simulink model "topfft"  (Simulink 7.6)
settings: Solver=FixedStepDiscrete  StartTime=0.0  StopTime=800  RelTol=1e-3
InitFcn:
  | %% DSPBuilder Start
  | alt_dspbuilder_update_model(bdroot)
  | %% DSPBuilder End
undefined symbols (not defined in the file): DSPBuilder_topfft_import, fft_stream
libraries: allblocks_alteradspbuilder2 x18, dspsrcs4 x4, simulink x3, megacorefunctions_alteradspbuilder2 x1
settings Model: Creator=lkong  LastModifiedBy=akarapet
settings OptimizationCC: InlineInvariantSignals=on  InitFltsAndDblsToZero=on
settings DebuggingCC: SaveWithParameterizedLinksMsg=none  SignalResolutionControl=TryResolveAllWithWarning  SolverPrmCheckMsg=none  MultiTaskDSMMsg=warning  MultiTaskCondExecSysMsg=none  StrictBusMsg=Warning
settings HardwareCC: TargetUnknown=on
settings RTWCC: IncludeERTFirstTime=on
settings GRTTargetCC: TargetFcnLib=ansi_tfl_tmw.mat

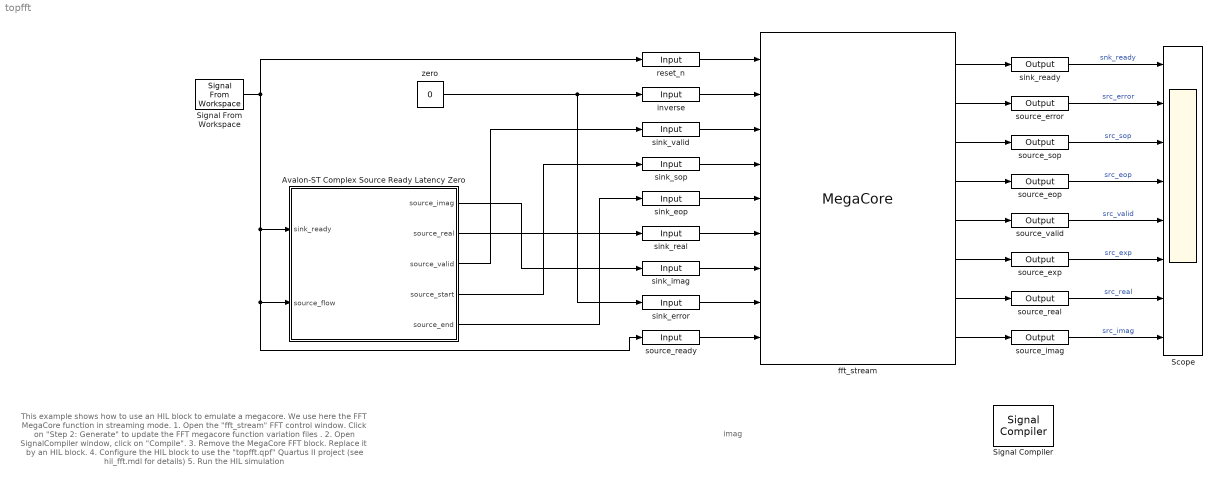
== system topfft ==
  note: imag
  note: This example shows how to use an HIL block to emulate a megacore.
      | We use here the FFT MegaCore function in streaming mode.
      | 1. Open the "fft_stream" FFT control window. Click on "Step 2: Generate" to update the FFT megacore function variation files .
      | 2. Open SignalCompiler window, click on "Compile".
      | 3. Remove the MegaCore FFT block. Replace it by an HIL block.
      | 4. Configure the HIL block to use the "topfft.qpf" Quartus II project (see hil_fft.mdl for details)
      | 5. Run the HIL simulation
  Avalon-ST Complex Source Ready Latency Zero : Subsystem  mask{datastring=[1:32], sopstring=[1 zeros(1,63)], eopstring=[zeros(1,63) 1], finaloption=Cyclic Repetition}
      mask prompts: datastring "Complex Data"; sopstring "Start of Packet"; eopstring "End of Packet"; finaloption "Form output after final data by"
      mask StyleString: edit,edit,edit,popup(Cyclic Repetition)
      mask Display:
      | port_label('input',1,'sink_ready');
      | port_label('input',2,'source_flow');
      | 
      | port_label('output',1,'source_imag');
      | port_label('output',2,'source_real');
      | port_label('output',3,'source_valid');
      | port_label('output',4,'source_start');
      | port_label('output',5,'source_end');
      | 
      | disp(&1);
  Scope : Scope  NumInputPorts=8
      settings: TimeRange=800  YMin=0~0~-1~-4~-20~-10~0~0  YMax=1~1~1~0~30~70~1~1
  Signal Compiler : allblocks_alteradspbuilder2/Signal Compiler  DeviceFamily=Cyclone III  DeviceName=EP3C120F780C7  EnableSignalTap=off  SignalTapDepth=128  UseBoardBlock=off  StpUseDefaultClock=on  StpClock=Clock  ExportDir=/data/akarapet/qshell_linux64_test/p4/dsp_builder/dsp_builder2/Documentation/DesignExamples/Tutorials/HIL/FFT
  Signal From Workspace : dspsrcs4/Signal From Workspace  SystemSampleTime=-1  X=[0 1]  Ts=1  nsamps=1  OutputAfterFinalValue=Holding final value  ignoreOrWarnInputAndFrameLengths=off
  fft_stream : megacorefunctions_alteradspbuilder2/MegaCore  entityName=fft_stream_import  inNames=reset_n inverse sink_valid sink_sop sink_eop sink_real sink_imag sink_error source_ready  inBwls="1   1   1   1   1  16  16   2   1"  inBwrs="0  0  0  0  0  0  0  0  0"  inTypes=b b b b b s s s b  inDelayed="0  1  1  1  1  1  1  1  1"  outNames=sink_ready source_error source_sop source_eop source_valid source_exp source_real source_imag  outBwls="1   2   1   1   1   6  16  16"  outBwrs="0  0  0  0  0  0  0  0"  outTypes=b s b b b s s s  xmlmapfile=/data/akarapet/qshell_linux64_test/acds/quartus/dsp_builder/lib/SimgenCMap.xml  is_megacore=on  use_dynamic_feedthrough_data=on  use_alphabetical_port_ordering=off  vofile=DSPBuilder_topfft_import/fft_stream.vo  n_input_port=9  n_output_port=8  core_dir=/data/akarapet/qshell_linux64_test/acds/ip/altera/fft/lib/ip_toolbench  core_name=fft  clockname=clk  flow_dir=/data/akarapet/qshell_linux64_test/acds/ip/altera/fft/lib/../../common/ip_toolbench/v1.3.0/bin  NewVariation=off  VhdlVariationDate=19-Jun-2013 09:53:44  VhdlVariationName=/data/akarapet/qshell_linux64_test/p4/dsp_builder/dsp_builder2/Documentation/DesignExamples/Tutorials/HIL/FFT/DSPBuilder_topfft_import/fft_stream.vhd  use_systemC_model=off  wizard=fft  inptype=bbbbbsssb  outptype=bsbbbsss  allowFloatingPointOverride=off
  inverse : allblocks_alteradspbuilder2/Input  iofile=/data/akarapet/qshell_linux64_test/p4/dsp_builder/dsp_builder2/Documentation/DesignExamples/Tutorials/HIL/FFT/tb_topfft/topfft_inverse.salt  BusType=Single Bit  bwl=1  bwr=0  SpecifyClock=off  PORTTYPE=Input  externalType=Inferred  allowFloatingPointOverride=on  logOutputs=off
  reset_n : allblocks_alteradspbuilder2/Input  iofile=/data/akarapet/qshell_linux64_test/p4/dsp_builder/dsp_builder2/Documentation/DesignExamples/Tutorials/HIL/FFT/tb_topfft/topfft_reset%5Fn.salt  BusType=Single Bit  bwl=1  bwr=0  SpecifyClock=off  PORTTYPE=Input  externalType=Inferred  allowFloatingPointOverride=on  logOutputs=off
  sink_eop : allblocks_alteradspbuilder2/Input  iofile=/data/akarapet/qshell_linux64_test/p4/dsp_builder/dsp_builder2/Documentation/DesignExamples/Tutorials/HIL/FFT/tb_topfft/topfft_sink%5Feop.salt  BusType=Single Bit  bwl=1  bwr=0  SpecifyClock=off  PORTTYPE=Input  externalType=Inferred  allowFloatingPointOverride=on  logOutputs=off
  sink_error : allblocks_alteradspbuilder2/Input  iofile=/data/akarapet/qshell_linux64_test/p4/dsp_builder/dsp_builder2/Documentation/DesignExamples/Tutorials/HIL/FFT/tb_topfft/topfft_sink%5Ferror.salt  BusType=Signed Integer  bwl=2  bwr=0  SpecifyClock=off  PORTTYPE=Input  externalType=Inferred  allowFloatingPointOverride=on  logOutputs=off
  sink_imag : allblocks_alteradspbuilder2/Input  iofile=/data/akarapet/qshell_linux64_test/p4/dsp_builder/dsp_builder2/Documentation/DesignExamples/Tutorials/HIL/FFT/tb_topfft/topfft_sink%5Fimag.salt  BusType=Signed Integer  bwl=16  bwr=0  SpecifyClock=off  PORTTYPE=Input  externalType=Inferred  allowFloatingPointOverride=on  logOutputs=off
  sink_ready : allblocks_alteradspbuilder2/Output  iofile=/data/akarapet/qshell_linux64_test/p4/dsp_builder/dsp_builder2/Documentation/DesignExamples/Tutorials/HIL/FFT/tb_topfft/topfft_sink%5Fready.capture  BusType=Single Bit  bwl=1  bwr=0  externalType=Inferred  PORTTYPE=Output  allowFloatingPointOverride=on  logOutputs=off
  sink_real : allblocks_alteradspbuilder2/Input  iofile=/data/akarapet/qshell_linux64_test/p4/dsp_builder/dsp_builder2/Documentation/DesignExamples/Tutorials/HIL/FFT/tb_topfft/topfft_sink%5Freal.salt  BusType=Signed Integer  bwl=16  bwr=0  SpecifyClock=off  PORTTYPE=Input  externalType=Inferred  allowFloatingPointOverride=on  logOutputs=off
  sink_sop : allblocks_alteradspbuilder2/Input  iofile=/data/akarapet/qshell_linux64_test/p4/dsp_builder/dsp_builder2/Documentation/DesignExamples/Tutorials/HIL/FFT/tb_topfft/topfft_sink%5Fsop.salt  BusType=Single Bit  bwl=1  bwr=0  SpecifyClock=off  PORTTYPE=Input  externalType=Inferred  allowFloatingPointOverride=on  logOutputs=off
  sink_valid : allblocks_alteradspbuilder2/Input  iofile=/data/akarapet/qshell_linux64_test/p4/dsp_builder/dsp_builder2/Documentation/DesignExamples/Tutorials/HIL/FFT/tb_topfft/topfft_sink%5Fvalid.salt  BusType=Single Bit  bwl=1  bwr=0  SpecifyClock=off  PORTTYPE=Input  externalType=Inferred  allowFloatingPointOverride=on  logOutputs=off
  source_eop : allblocks_alteradspbuilder2/Output  iofile=/data/akarapet/qshell_linux64_test/p4/dsp_builder/dsp_builder2/Documentation/DesignExamples/Tutorials/HIL/FFT/tb_topfft/topfft_source%5Feop.capture  BusType=Single Bit  bwl=1  bwr=0  externalType=Inferred  PORTTYPE=Output  allowFloatingPointOverride=on  logOutputs=off
  source_error : allblocks_alteradspbuilder2/Output  iofile=/data/akarapet/qshell_linux64_test/p4/dsp_builder/dsp_builder2/Documentation/DesignExamples/Tutorials/HIL/FFT/tb_topfft/topfft_source%5Ferror.capture  BusType=Signed Integer  bwl=2  bwr=0  externalType=Inferred  PORTTYPE=Output  allowFloatingPointOverride=on  logOutputs=off
  source_exp : allblocks_alteradspbuilder2/Output  iofile=/data/akarapet/qshell_linux64_test/p4/dsp_builder/dsp_builder2/Documentation/DesignExamples/Tutorials/HIL/FFT/tb_topfft/topfft_source%5Fexp.capture  BusType=Signed Integer  bwl=6  bwr=0  externalType=Inferred  PORTTYPE=Output  allowFloatingPointOverride=on  logOutputs=off
  source_imag : allblocks_alteradspbuilder2/Output  iofile=/data/akarapet/qshell_linux64_test/p4/dsp_builder/dsp_builder2/Documentation/DesignExamples/Tutorials/HIL/FFT/tb_topfft/topfft_source%5Fimag.capture  BusType=Signed Integer  bwl=16  bwr=0  externalType=Inferred  PORTTYPE=Output  allowFloatingPointOverride=on  logOutputs=off
  source_ready : allblocks_alteradspbuilder2/Input  iofile=/data/akarapet/qshell_linux64_test/p4/dsp_builder/dsp_builder2/Documentation/DesignExamples/Tutorials/HIL/FFT/tb_topfft/topfft_source%5Fready.salt  BusType=Single Bit  bwl=1  bwr=0  SpecifyClock=off  PORTTYPE=Input  externalType=Inferred  allowFloatingPointOverride=on  logOutputs=off
  source_real : allblocks_alteradspbuilder2/Output  iofile=/data/akarapet/qshell_linux64_test/p4/dsp_builder/dsp_builder2/Documentation/DesignExamples/Tutorials/HIL/FFT/tb_topfft/topfft_source%5Freal.capture  BusType=Signed Integer  bwl=16  bwr=0  externalType=Inferred  PORTTYPE=Output  allowFloatingPointOverride=on  logOutputs=off
  source_sop : allblocks_alteradspbuilder2/Output  iofile=/data/akarapet/qshell_linux64_test/p4/dsp_builder/dsp_builder2/Documentation/DesignExamples/Tutorials/HIL/FFT/tb_topfft/topfft_source%5Fsop.capture  BusType=Single Bit  bwl=1  bwr=0  externalType=Inferred  PORTTYPE=Output  allowFloatingPointOverride=on  logOutputs=off
  source_valid : allblocks_alteradspbuilder2/Output  iofile=/data/akarapet/qshell_linux64_test/p4/dsp_builder/dsp_builder2/Documentation/DesignExamples/Tutorials/HIL/FFT/tb_topfft/topfft_source%5Fvalid.capture  BusType=Single Bit  bwl=1  bwr=0  externalType=Inferred  PORTTYPE=Output  allowFloatingPointOverride=on  logOutputs=off
  zero : Constant  Value=0
  wires:
  zero/1 -> sink_error/1, inverse/1
  sink_imag/1 -> fft_stream/7
  sink_real/1 -> fft_stream/6
  inverse/1 -> fft_stream/2
  sink_sop/1 -> fft_stream/4
  fft_stream/4 -> source_eop/1
  fft_stream/2 -> source_error/1
  fft_stream/6 -> source_exp/1
  fft_stream/8 -> source_imag/1
  source_eop/1 -> Scope/4  "src_eop"
  source_error/1 -> Scope/2  "src_error"
  source_exp/1 -> Scope/6  "src_exp"
  source_imag/1 -> Scope/8  "src_imag"
  source_real/1 -> Scope/7  "src_real"
  source_sop/1 -> Scope/3  "src_sop"
  source_valid/1 -> Scope/5  "src_valid"
  sink_valid/1 -> fft_stream/3
  fft_stream/3 -> source_sop/1
  fft_stream/7 -> source_real/1
  source_ready/1 -> fft_stream/9
  fft_stream/1 -> sink_ready/1
  sink_error/1 -> fft_stream/8
  sink_eop/1 -> fft_stream/5
  Signal From Workspace/1 -> source_ready/1, Avalon-ST Complex Source Ready Latency Zero/2(source_flow), Avalon-ST Complex Source Ready Latency Zero/1(sink_ready), reset_n/1
  fft_stream/5 -> source_valid/1
  reset_n/1 -> fft_stream/1
  sink_ready/1 -> Scope/1  "snk_ready"
  Avalon-ST Complex Source Ready Latency Zero/1(source_imag) -> sink_imag/1
  Avalon-ST Complex Source Ready Latency Zero/2(source_real) -> sink_real/1
  Avalon-ST Complex Source Ready Latency Zero/4(source_start) -> sink_sop/1
  Avalon-ST Complex Source Ready Latency Zero/5(source_end) -> sink_eop/1
  Avalon-ST Complex Source Ready Latency Zero/3(source_valid) -> sink_valid/1

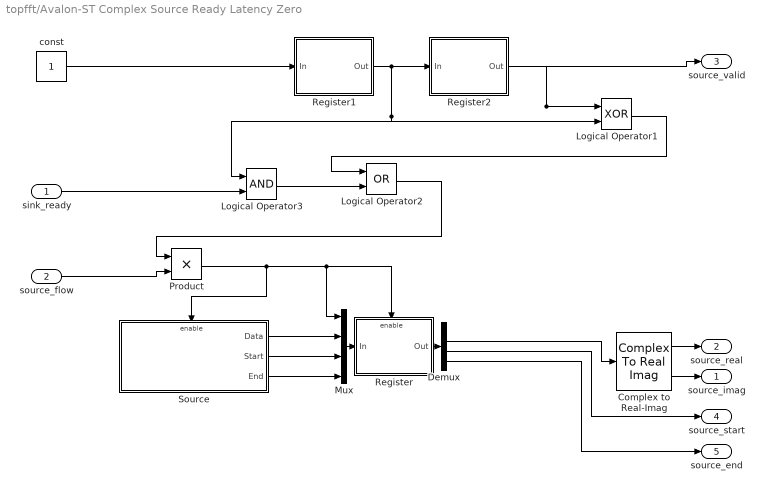
== system topfft/Avalon-ST Complex Source Ready Latency Zero ==
  sink_ready : Inport
  source_flow : Inport  Port=2
  Complex to Real-Imag : ComplexToRealImag
  Demux : Demux
  Logical Operator1 : Logic  Operator=XOR  AllPortsSameDT=off  OutDataTypeStr=boolean
  Logical Operator2 : Logic  Operator=OR  AllPortsSameDT=off  OutDataTypeStr=boolean
  Logical Operator3 : Logic  AllPortsSameDT=off  OutDataTypeStr=boolean
  Mux : Mux
  Product : Product  RndMeth=Zero
  Register : Subsystem  TreatAsAtomicUnit=on
  Register1 : Subsystem  TreatAsAtomicUnit=on
  Register2 : Subsystem  TreatAsAtomicUnit=on
  Source : Subsystem  TreatAsAtomicUnit=on  mask{datastring=datastring, sopstring=sopstring, eopstring=eopstring}
      mask prompts: datastring "Complex Data"; sopstring "Start of Packet"; eopstring "End of Packet"
  const : Constant
  source_imag : Outport
  source_real : Outport  Port=2
  source_valid : Outport  Port=3
  source_start : Outport  Port=4
  source_end : Outport  Port=5
  wires:
  Demux/4 -> source_end/1
  Demux/3 -> source_start/1
  Demux/2 -> Complex to Real-Imag/1
  Source/1(Data) -> Mux/2
  Source/2(Start) -> Mux/3
  Source/3(End) -> Mux/4
  Complex to Real-Imag/2 -> source_imag/1
  Complex to Real-Imag/1 -> source_real/1
  Register/1(Out) -> Demux/1
  Mux/1 -> Register/1(In)
  Product/1 -> Source/Enable, Mux/1, Register/Enable
  source_flow/1 -> Product/2
  Register1/1(Out) -> Register2/1(In), Logical Operator1/2, Logical Operator3/1
  const/1 -> Register1/1(In)
  Register2/1(Out) -> Logical Operator1/1, source_valid/1
  sink_ready/1 -> Logical Operator3/2
  Logical Operator1/1 -> Logical Operator2/1
  Logical Operator2/1 -> Product/1
  Logical Operator3/1 -> Logical Operator2/2

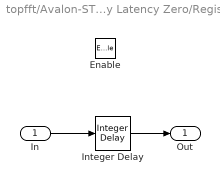
== system topfft/Avalon-ST Complex Source Ready Latency Zero/Register ==
  In : Inport
  Enable : EnablePort
  Integer Delay : simulink/Discrete/Integer Delay  NumDelays=1  InputProcessing=Inherited  vinit=0.0  samptime=-1
  Out : Outport
  wires:
  Integer Delay/1 -> Out/1
  In/1 -> Integer Delay/1

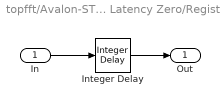
== system topfft/Avalon-ST Complex Source Ready Latency Zero/Register1 ==
  In : Inport
  Integer Delay : simulink/Discrete/Integer Delay  NumDelays=1  InputProcessing=Inherited  vinit=0.0  samptime=-1
  Out : Outport
  wires:
  Integer Delay/1 -> Out/1
  In/1 -> Integer Delay/1

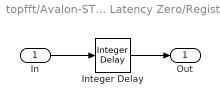
== system topfft/Avalon-ST Complex Source Ready Latency Zero/Register2 ==
  In : Inport
  Integer Delay : simulink/Discrete/Integer Delay  NumDelays=1  InputProcessing=Inherited  vinit=0.0  samptime=-1
  Out : Outport
  wires:
  Integer Delay/1 -> Out/1
  In/1 -> Integer Delay/1

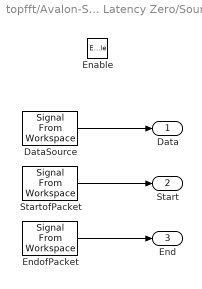
== system topfft/Avalon-ST Complex Source Ready Latency Zero/Source ==
  Enable : EnablePort
  DataSource : dspsrcs4/Signal From Workspace  SystemSampleTime=-1  X=datastring  Ts=-1  nsamps=1  OutputAfterFinalValue=Cyclic repetition  ignoreOrWarnInputAndFrameLengths=off
  EndofPacket : dspsrcs4/Signal From Workspace  SystemSampleTime=-1  X=eopstring  Ts=-1  nsamps=1  OutputAfterFinalValue=Cyclic repetition  ignoreOrWarnInputAndFrameLengths=off
  StartofPacket : dspsrcs4/Signal From Workspace  SystemSampleTime=-1  X=sopstring  Ts=-1  nsamps=1  OutputAfterFinalValue=Cyclic repetition  ignoreOrWarnInputAndFrameLengths=off
  Data : Outport
  Start : Outport  Port=2
  End : Outport  Port=3
  wires:
  EndofPacket/1 -> End/1
  StartofPacket/1 -> Start/1
  DataSource/1 -> Data/1
